simulink library "Hot_Water_Consumption_EN13203"  (Simulink 7.6)
settings: Solver=ode45  StartTime=0.0  StopTime=10.0  RelTol=1e-3
settings Model: Creator=lena.frank  LastModifiedBy=awohlfei

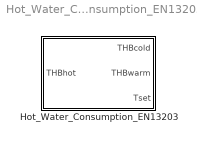
== system Hot_Water_Consumption_EN13203 ==
  Hot_Water_Consumption_EN13203 : Subsystem
      mask Display: plot(0,0,140,130,[70,76,78,63,65,70,70,10],[80,78,74,74,78,80,100,100],[23,23,20,10],[43,47,50,50],[10,10,20,28,30,10],[30,20,20,23,30,30],[22,17],[54,54],[20,20],[54,50],[90,90,50,50],[10,-0,-0,10],[63,64],[60,72],[61,62],[38,50],[60,61],[13,27],[90,85,81,76,70,65,59,54,50],[6,4,6,4,6,4,5,3,5],[68,69],[56,68],[68,68],[32,44],[67,67],[13,23],[73,73],[61,71],[73,73],[43,52],[74,73],[21,36],[78,77],[56,67],[79,79],[34,45],[78,77],[9,23],[82,81],[14,26])

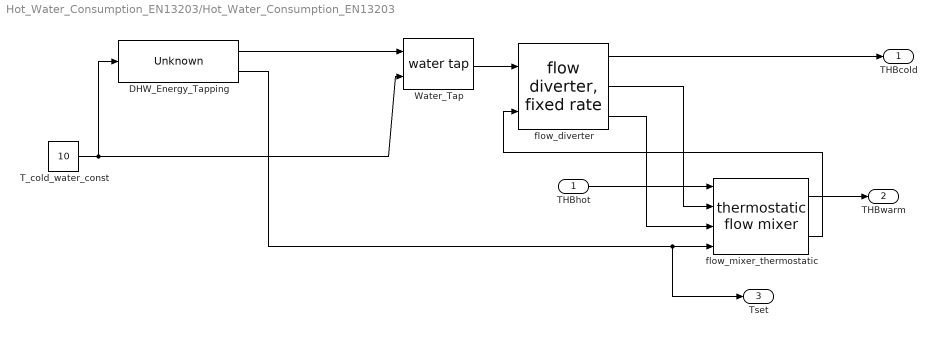
== system Hot_Water_Consumption_EN13203/Hot_Water_Consumption_EN13203 ==
  THBhot : Inport
  DHW_Energy_Tapping : Reference  mdot_nom=0.1  times=[7 12 19]*3600  energies=[4 2 4]*3600000  dT_set=[35 35 35]  coeffs=[1 1 1]
  T_cold_water_const : Constant  Value=10
  Water_Tap : Reference  SystemSampleTime=-1  dia=0.02  p=2e5
  flow_diverter : Reference  SystemSampleTime=-1
  flow_mixer_thermostatic : Reference  SystemSampleTime=-1  t=10
  THBcold : Outport  InitialOutput=0
  THBwarm : Outport  Port=2
  Tset : Outport  Port=3  InitialOutput=0
  wires:
  DHW_Energy_Tapping/2 -> flow_mixer_thermostatic/4, Tset/1
  flow_diverter/3 -> flow_mixer_thermostatic/3
  flow_diverter/2 -> flow_mixer_thermostatic/2
  flow_diverter/1 -> THBcold/1
  THBhot/1 -> flow_mixer_thermostatic/1
  flow_mixer_thermostatic/1 -> THBwarm/1
  flow_mixer_thermostatic/2 -> flow_diverter/2
  Water_Tap/1 -> flow_diverter/1
  T_cold_water_const/1 -> Water_Tap/2, DHW_Energy_Tapping/1
  DHW_Energy_Tapping/1 -> Water_Tap/1
